simulink model "Sim_Plant_x"  (R2017a)
settings: Solver=ode3  StartTime=0.0  StopTime=5  FixedStep=1/50  RelTol=1e-3  EnableMultiTasking=on
values from neighbouring files (symbols this model uses):
  mQ = 0.5645    [LG_ID_ss_Model.m]
undefined symbols (not defined in the file or in its folder): Kd_x, Kd_z, Ki_z, Kp_x, Kp_z, magnitude
libraries: simulink x1
settings Model: Creator=GeoLee  LastModifiedBy=gmh_n
settings DataIOCC: LimitDataPoints=on  SaveFormat=Array
settings OptimizationCC: ExpressionDepthLimit=2147483647  LifeSpan=inf
settings DebuggingCC: UnderspecifiedInitializationDetection=Classic  MergeDetectMultiDrivingBlocksExec=none  SolverPrmCheckMsg=warning  StateNameClashWarn=warning  SFUnexpectedBacktrackingDiag=warning  SFNoUnconditionalDefaultTransitionDiag=warning  SFExecutionAtInitializationDiag=none
settings HardwareCC: ProdBitPerPointer=32  ProdBitPerSizeT=32  ProdBitPerPtrDiffT=32  ProdLargestAtomicFloat=None  ProdIntDivRoundTo=Undefined  ProdEndianess=Unspecified  ProdWordSize=32  ProdHWDeviceType=32-bit Generic
settings ModelReferenceCC: PropagateSignalLabelsOutOfModel=off
settings GRTTargetCC: TargetLangStandard=C89/C90 (ANSI)  GeneratePreprocessorConditionals=Disable all
settings ConfigComp: CovMetricSettings=dw  CovHtmlReporting=on  CovSaveCumulativeToWorkspaceVar=on  CovSaveSingleToWorkspaceVar=on  CovExternalEMLEnable=off

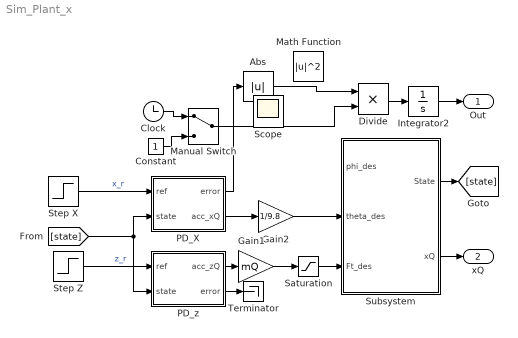
== system Sim_Plant_x ==
  Abs : Abs
  Clock : Clock
  Constant : Constant
  Divide : Product  Inputs=**
  Gain1 : Gain  Gain=mQ
  Gain2 : Gain  Gain=1/9.8
  Integrator2 : Integrator
  Manual Switch : ManualSwitch
  Math Function : Math  Operator=magnitude^2  SaturateOnIntegerOverflow=on
  PD_X : Subsystem
  PD_z : Subsystem
  Saturation : Saturate  UpperLimit=10  LowerLimit=-0.5645*9.8
  Step X : Step  After=0.2  SampleTime=0
  Step Z : Step  After=0  SampleTime=0
  Subsystem : Subsystem
  Terminator : Terminator
  Out : Outport
  xQ : Outport  Port=2
  Scope : Scope
  wires:
  Subsystem/1(State) -> [state]
  [state] -> PD_z/2(state), PD_X/2(state)
  Step Z/1 -> PD_z/1(ref)  "z_r"
  PD_z/1(acc_zQ) -> Gain1/1
  Saturation/1 -> Subsystem/3(Ft_des)
  Integrator2/1 -> Out/1
  Divide/1 -> Integrator2/1
  Manual Switch/1 -> Divide/2
  PD_z/2(error) -> Terminator/1
  PD_X/2(acc_xQ) -> Gain2/1
  Step X/1 -> PD_X/1(ref)  "x_r"
  PD_X/1(error) -> Abs/1
  Gain1/1 -> Saturation/1
  Subsystem/2(xQ) -> xQ/1
  Gain2/1 -> Subsystem/2(theta_des)
  Clock/1 -> Manual Switch/1
  Constant/1 -> Manual Switch/2
  Abs/1 -> Divide/1

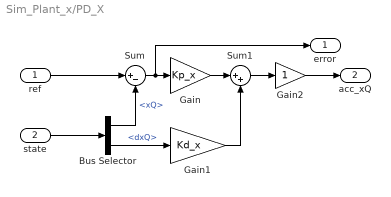
== system Sim_Plant_x/PD_X ==
  ref : Inport
  state : Inport  Port=2
  Bus Selector : BusSelector  OutputSignals=xQ,dxQ
  Gain : Gain  Gain=Kp_x
  Gain1 : Gain  Gain=Kd_x
  Gain2 : Gain
  Sum : Sum  Inputs=|+-
  Sum1 : Sum  Inputs=|++
  error : Outport
  acc_xQ : Outport  Port=2
  wires:
  Gain2/1 -> acc_xQ/1
  Gain1/1 -> Sum1/2
  Sum1/1 -> Gain2/1
  Gain/1 -> Sum1/1
  Bus Selector/2 -> Gain1/1  "<dxQ>"
  state/1 -> Bus Selector/1
  ref/1 -> Sum/1
  Bus Selector/1 -> Sum/2  "<xQ>"
  Sum/1 -> error/1, Gain/1

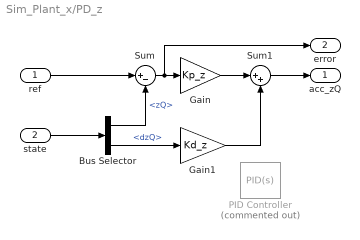
== system Sim_Plant_x/PD_z ==
  ref : Inport
  state : Inport  Port=2
  Bus Selector : BusSelector  OutputSignals=zQ,dzQ
  Gain : Gain  Gain=Kp_z
  Gain1 : Gain  Gain=Kd_z
  PID Controller : simulink/Continuous/PID Controller  Commented=on  Controller=PID  TimeDomain=Continuous-time  SampleTime=-1  IntegratorMethod=Forward Euler  FilterMethod=Forward Euler  Form=Parallel  UseFilter=on  ControllerParametersSource=internal  P=Kp_z  I=Ki_z  D=0  N=100  InitialConditionSource=internal  InitialConditionForIntegrator=0  InitialConditionForFilter=0  ExternalReset=none  LimitOutput=off  UpperSaturationLimit=inf  LowerSaturationLimit=-inf  LinearizeAsGain=on  AntiWindupMode=none  Kb=1  TrackingMode=off  Kt=1  PParamMin=[]  PParamMax=[]  IParamMin=[]  IParamMax=[]  DParamMin=[]  DParamMax=[]  NParamMin=[]  NParamMax=[]  KbParamMin=[]  KbParamMax=[]  KtParamMin=[]  KtParamMax=[]  POutMin=[]  POutMax=[]  IOutMin=[]  IOutMax=[]  DOutMin=[]  DOutMax=[]  NOutMin=[]  NOutMax=[]  KbOutMin=[]  KbOutMax=[]  KtOutMin=[]  KtOutMax=[]  IntegratorOutMin=[]  IntegratorOutMax=[]  FilterOutMin=[]  FilterOutMax=[]  SumOutMin=[]  SumOutMax=[]  SumI1OutMin=[]  SumI1OutMax=[]  SumI2OutMin=[]  SumI2OutMax=[]  SumI3OutMin=[]  SumI3OutMax=[]  SumDOutMin=[]  SumDOutMax=[]  SaturationOutMin=[]  SaturationOutMax=[]  IntegratorContinuousStateAttributes=''  IntegratorStateMustResolveToSignalObject=off  IntegratorRTWStateStorageClass=Auto  FilterContinuousStateAttributes=''  FilterStateMustResolveToSignalObject=off  FilterRTWStateStorageClass=Auto  DifferentiatorICPrevScaledInput=0  DifferentiatorOutMin=[]  DifferentiatorOutMax=[]  InitialConditionSetting=State (most efficient)
  Sum : Sum  Inputs=|+-
  Sum1 : Sum  Inputs=|++
  acc_zQ : Outport
  error : Outport  Port=2
  wires:
  Gain1/1 -> Sum1/2
  Sum1/1 -> acc_zQ/1
  Gain/1 -> Sum1/1
  Bus Selector/2 -> Gain1/1  "<dzQ>"
  state/1 -> Bus Selector/1
  Sum/1 -> Gain/1, error/1
  ref/1 -> Sum/1
  Bus Selector/1 -> Sum/2  "<zQ>"

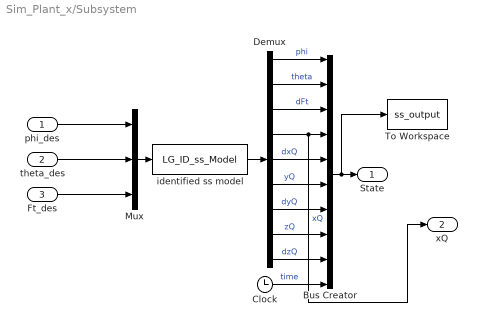
== system Sim_Plant_x/Subsystem ==
  phi_des : Inport
  theta_des : Inport  Port=2
  Ft_des : Inport  Port=3
  Bus Creator : BusCreator  Inputs=10
  Clock : Clock
  Demux : Demux  Outputs=9
  Mux : Mux  Inputs=3
  To Workspace : ToWorkspace  VariableName=ss_output  SampleTime=-1
  identified ss model : S-Function  FunctionName=LG_ID_ss_Model  SFunctionDeploymentMode=off  EnableBusSupport=off
  State : Outport
  xQ : Outport  Port=2
  wires:
  Clock/1 -> Bus Creator/10  "time"
  identified ss model/1 -> Demux/1
  Mux/1 -> identified ss model/1
  Ft_des/1 -> Mux/3
  phi_des/1 -> Mux/1
  theta_des/1 -> Mux/2
  Demux/6 -> Bus Creator/6  "yQ"
  Demux/7 -> Bus Creator/7  "dyQ"
  Demux/4 -> xQ/1, Bus Creator/4  "xQ"
  Demux/9 -> Bus Creator/9  "dzQ"
  Demux/5 -> Bus Creator/5  "dxQ"
  Demux/1 -> Bus Creator/1  "phi"
  Demux/3 -> Bus Creator/3  "dFt"
  Demux/2 -> Bus Creator/2  "theta"
  Demux/8 -> Bus Creator/8  "zQ"
  Bus Creator/1 -> To Workspace/1, State/1
